simulink model "MultiEffectEvaporator_Forward"  (R2024a)
settings: Solver=VariableStepAuto  StartTime=0.0  StopTime=50  MaxStep=0.05  RelTol=1e-3
libraries: slpidlib x3
settings Model: Creator=tmlouw  LastModifiedBy=tmlouw

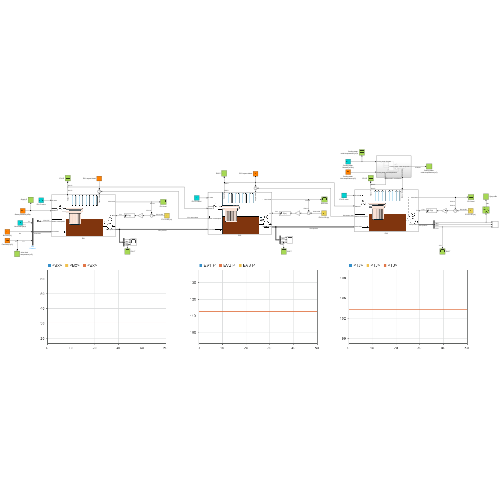
[thumbnail: Simulink's stored preview of the top-level diagram]
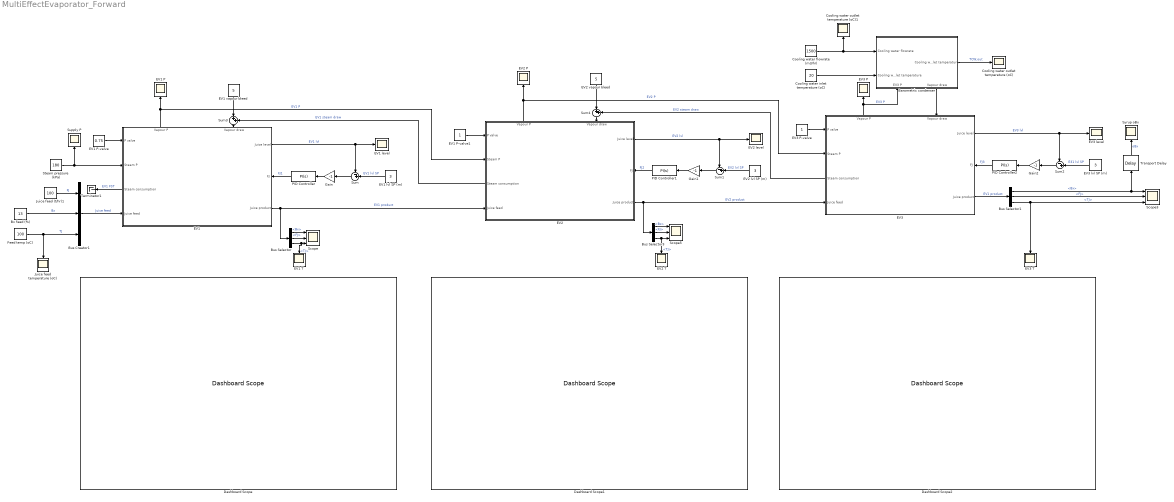
== system MultiEffectEvaporator_Forward ==
  Barometric condenser : Subsystem
      settings: PortSchema="{\"entries\":[{\"content\":{\"sides\":[{\"content\":{\"connectorIds\":[\"In1\",\"In2\"]},\"type\":\"ConnectorPlacement.EquallySpacedRectSide\",\"uuid\":\"e5056713-d8d2-44cb-a01c-60287b02fa20\"},{\"content\":{\"connectorIds\":[\"Out1\"],\"side\":\"RIGHT\"},\"type\":\"ConnectorPlacement.EquallySpacedRectSide\",\"uuid\":\"75a49828-ba17-4d10-97f5-6b462429e837\"},{\"content\":{\"side\":\"TOP\"},\"type\":\"ConnectorPlacement.EquallySpacedRectSide\",\"uuid\":\"088b5e1d-8405-4455-9e05-b28295e853da\"},{\"content\":{\"connectorIds\":[\"In3\",\"Out2\"],\"side\":\"BOTTOM\"},\"type\":\"ConnectorPlacement.EquallySpacedRectSide\",\"uuid\":\"29e66075-be5c-4fc5-8b50-76bd472c32b2\"}]},\"type\":\"ConnectorPlacement.EquallySpacedConnector\",\"uuid\":\"8d291cf1-31f4-4e5b-a130-7090ea448cc4\"}],\"packageUris\":[\"http://schema.mathworks.com/mf0/Connector/R2020b\"],\"version\":\"1.0\"}"
  Bus Creator1 : BusCreator  Inputs=3
  Bus Selector : BusSelector  OutputSignals=Bx,FJ,TJ
  Bus Selector1 : BusSelector  OutputSignals=Bx,FJ,TJ
  Bus Selector3 : BusSelector  OutputSignals=Bx,FJ,TJ
  Bx feed (%) : Constant  Value=13
  Cooling water flowrate (m3/hr) : Constant  Value=1500
  Cooling water inlet temperature (oC) : Constant  Value=20
  Cooling water outlet temperature (oC) : Scope
  Cooling water outlet temperature (oC)1 : Scope
  Dashboard Scope : DashboardScope
  Dashboard Scope1 : DashboardScope
  Dashboard Scope2 : DashboardScope
  EV1 : Subsystem
      settings: PortSchema="{\"entries\":[{\"content\":{\"sides\":[{\"content\":{\"connectorIds\":[\"In1\",\"In2\",\"Out4\",\"In3\"]},\"type\":\"ConnectorPlacement.EquallySpacedRectSide\",\"uuid\":\"23f23739-dcb1-4c27-bdfa-9a4fab3adfb4\"},{\"content\":{\"connectorIds\":[\"Out1\",\"In5\",\"Out2\"],\"side\":\"RIGHT\"},\"type\":\"ConnectorPlacement.EquallySpacedRectSide\",\"uuid\":\"36d72309-34f0-453c-bd76-e3ebc7b1c9b0\"},{\"content\":{\"connectorIds\":[\"Out3\",\"In4\"],\"side\":\"TOP\"},\"type\":\"ConnectorPlacement.EquallySpacedRectSide\",\"uuid\":\"a2c1fcb6-fda4-47d3-b526-f27431a4eb07\"},{\"content\":{\"side\":\"BOTTOM\"},\"type\":\"ConnectorPlacement.EquallySpacedRectSide\",\"uuid\":\"52c37164-7db0-4f32-b080-c60396f400a7\"}]},\"type\":\"ConnectorPlacement.EquallySpacedConnector\",\"uuid\":\"33257158-25c1-436c-a188-64f6424e9d36\"}],\"packageUris\":[\"http://schema.mathworks.com/mf0/Connector/R2020b\"],\"version\":\"1.0\"}"
      mask Display: image('MaskForward.png');
  EV1 P : Scope
  EV1 P-valve : Constant  Value=0.75
  EV1 P-valve1 : Constant
  EV1 T : Scope
  EV1 level : Scope
  EV1 lvl SP (m) : Constant  Value=3
  EV1 vapour bleed : Constant  Value=5
  EV2 : Subsystem
      settings: PortSchema="{\"entries\":[{\"content\":{\"sides\":[{\"content\":{\"connectorIds\":[\"In1\",\"In2\",\"Out4\",\"In3\"]},\"type\":\"ConnectorPlacement.EquallySpacedRectSide\",\"uuid\":\"23f23739-dcb1-4c27-bdfa-9a4fab3adfb4\"},{\"content\":{\"connectorIds\":[\"Out1\",\"In5\",\"Out2\"],\"side\":\"RIGHT\"},\"type\":\"ConnectorPlacement.EquallySpacedRectSide\",\"uuid\":\"36d72309-34f0-453c-bd76-e3ebc7b1c9b0\"},{\"content\":{\"connectorIds\":[\"Out3\",\"In4\"],\"side\":\"TOP\"},\"type\":\"ConnectorPlacement.EquallySpacedRectSide\",\"uuid\":\"a2c1fcb6-fda4-47d3-b526-f27431a4eb07\"},{\"content\":{\"side\":\"BOTTOM\"},\"type\":\"ConnectorPlacement.EquallySpacedRectSide\",\"uuid\":\"52c37164-7db0-4f32-b080-c60396f400a7\"}]},\"type\":\"ConnectorPlacement.EquallySpacedConnector\",\"uuid\":\"33257158-25c1-436c-a188-64f6424e9d36\"}],\"packageUris\":[\"http://schema.mathworks.com/mf0/Connector/R2020b\"],\"version\":\"1.0\"}"
      mask Display: image('MaskForward.png');
  EV2 P : Scope
  EV2 T : Scope
  EV2 level : Scope
  EV2 lvl SP (m) : Constant  Value=3
  EV2 vapour bleed : Constant  Value=5
  EV3 : Subsystem
      settings: PortSchema="{\"entries\":[{\"content\":{\"sides\":[{\"content\":{\"connectorIds\":[\"In1\",\"In2\",\"Out4\",\"In3\"]},\"type\":\"ConnectorPlacement.EquallySpacedRectSide\",\"uuid\":\"23f23739-dcb1-4c27-bdfa-9a4fab3adfb4\"},{\"content\":{\"connectorIds\":[\"Out1\",\"In5\",\"Out2\"],\"side\":\"RIGHT\"},\"type\":\"ConnectorPlacement.EquallySpacedRectSide\",\"uuid\":\"36d72309-34f0-453c-bd76-e3ebc7b1c9b0\"},{\"content\":{\"connectorIds\":[\"Out3\",\"In4\"],\"side\":\"TOP\"},\"type\":\"ConnectorPlacement.EquallySpacedRectSide\",\"uuid\":\"a2c1fcb6-fda4-47d3-b526-f27431a4eb07\"},{\"content\":{\"side\":\"BOTTOM\"},\"type\":\"ConnectorPlacement.EquallySpacedRectSide\",\"uuid\":\"52c37164-7db0-4f32-b080-c60396f400a7\"}]},\"type\":\"ConnectorPlacement.EquallySpacedConnector\",\"uuid\":\"33257158-25c1-436c-a188-64f6424e9d36\"}],\"packageUris\":[\"http://schema.mathworks.com/mf0/Connector/R2020b\"],\"version\":\"1.0\"}"
      mask Display: image('MaskForward.png');
  EV3 P : Scope
  EV3 P-valve : Constant
  EV3 T : Scope
  EV3 level : Scope
  EV3 lvl SP (m) : Constant  Value=3
  Feed temp (oC) : Constant  Value=100
  Gain : Gain  Gain=-1
  Gain1 : Gain  Gain=-1
  Gain2 : Gain  Gain=-1
  Juice feed temperature (oC) : Scope
  Juice feed (t/hr)1 : Constant  Value=100
  PID Controller : slpidlib/PID Controller  Controller=PI  Form=Parallel  TimeDomain=Continuous-time  UseExternalTs=off  SampleTime=-1  IntegratorMethod=Forward Euler  FilterMethod=Forward Euler  ControllerParametersSource=internal  P=1000  I=100  UseKiTs=off  D=0  UseExternalDerivativeSource=off  N=100  UseFilter=on  TunerSelectOption=Transfer Function Based (PID Tuner App)  InitialConditionSource=internal  InitialConditionForIntegrator=69.42  InitialConditionForFilter=0  DifferentiatorICPrevScaledInput=0  ExternalReset=none  TrackingMode=off  Kt=1  LimitOutput=on  SatLimitsSource=internal  UpperSaturationLimit=inf  LowerSaturationLimit=0  LinearizeAsGain=on  AntiWindupMode=none  Kb=1  LimitIntegrator=off  UpperIntegratorSaturationLimit=inf  LowerIntegratorSaturationLimit=-inf  POutMin=[]  POutMax=[]  IOutMin=[]  IOutMax=[]  DOutMin=[]  DOutMax=[]  NOutMin=[]  NOutMax=[]  SumOutMin=[]  SumOutMax=[]  SaturationOutMin=[]  SaturationOutMax=[]  PParamMin=[]  PParamMax=[]  IParamMin=[]  IParamMax=[]  DParamMin=[]  DParamMax=[]  NParamMin=[]  NParamMax=[]  KbParamMin=[]  KbParamMax=[]  KtParamMin=[]  KtParamMax=[]  KbOutMin=[]  KbOutMax=[]  KtOutMin=[]  KtOutMax=[]  IntegratorOutMin=[]  IntegratorOutMax=[]  FilterOutMin=[]  FilterOutMax=[]  SumI1OutMin=[]  SumI1OutMax=[]  SumI2OutMin=[]  SumI2OutMax=[]  SumI3OutMin=[]  SumI3OutMax=[]  SumI4OutMin=[]  SumI4OutMax=[]  SumDOutMin=[]  SumDOutMax=[]  DifferentiatorOutMin=[]  DifferentiatorOutMax=[]  FilterDiffOutCoefMin=[]  FilterDiffOutCoefMax=[]  ReciprocalOutMin=[]  ReciprocalOutMax=[]  SumDenOutMin=[]  SumDenOutMax=[]  SumNumOutMin=[]  SumNumOutMax=[]  DivideOutMin=[]  DivideOutMax=[]  UdiffTsProdOutMin=[]  UdiffTsProdOutMax=[]  NTsProdOutMin=[]  NTsProdOutMax=[]  UintegralTsProdOutMin=[]  UintegralTsProdOutMax=[]  UngainTsProdOutMin=[]  UngainTsProdOutMax=[]  ClampingZeroOutDataTypeStr=Inherit: Inherit via back propagation  ClampingZeroOutMin=[]  ClampingZeroOutMax=[]  FilterDenConstantOutDataTypeStr=Inherit: Inherit via back propagation  FilterDenConstantOutMin=[]  FilterDenConstantOutMax=[]  PCopyOutDataTypeStr=Inherit: Inherit via back propagation  PCopyOutMin=[]  PCopyOutMax=[]  NCopyOutDataTypeStr=Inherit: Inherit via back propagation  NCopyOutMin=[]  NCopyOutMax=[]  IntegratorContinuousStateAttributes=''  IntegratorStateMustResolveToSignalObject=off  IntegratorRTWStateStorageClass=Auto  FilterContinuousStateAttributes=''  FilterStateMustResolveToSignalObject=off  FilterRTWStateStorageClass=Auto  ParallelPVariant=InternalParameters  IdealPVariant=Disabled  IVariant=InternalParameters  DVariant=Disabled  IntegratorVariant=Continuous  SatVariant=Enabled  AWVariant=Passthrough  PCopyVariant=Disabled  TRVariant=Disabled  FdbkBlocksVariant=Forward  IdealPFdbkVariant=Disabled  SatFdbkVariant=Disabled  DerivativeFilterVariant=Disabled  NVariant=Disabled  NCopyVariant=Disabled_SignalSpec  FilterICVariant=Disabled  IntegratorICVariant=InternalICs  ExternalResetVariant=Disabled  TRSumVariant=Passthrough  SumFdbkVariant=Disabled  SumVariant=Sum_PI  TsampFilterVariant=InternalTs  TsampNgainVariant=Passthrough  TsampIntegralVariant=Disabled_SignalSpec  ExternalSaturationOutDataTypeStr=Inherit: Same as second input  DerivativeSourceVariant=Disabled
  PID Controller1 : slpidlib/PID Controller  Controller=PI  Form=Parallel  TimeDomain=Continuous-time  UseExternalTs=off  SampleTime=-1  IntegratorMethod=Forward Euler  FilterMethod=Forward Euler  ControllerParametersSource=internal  P=1000  I=100  UseKiTs=off  D=0  UseExternalDerivativeSource=off  N=100  UseFilter=on  TunerSelectOption=Transfer Function Based (PID Tuner App)  InitialConditionSource=internal  InitialConditionForIntegrator=43  InitialConditionForFilter=0  DifferentiatorICPrevScaledInput=0  ExternalReset=none  TrackingMode=off  Kt=1  LimitOutput=on  SatLimitsSource=internal  UpperSaturationLimit=inf  LowerSaturationLimit=0  LinearizeAsGain=on  AntiWindupMode=none  Kb=1  LimitIntegrator=off  UpperIntegratorSaturationLimit=inf  LowerIntegratorSaturationLimit=-inf  POutMin=[]  POutMax=[]  IOutMin=[]  IOutMax=[]  DOutMin=[]  DOutMax=[]  NOutMin=[]  NOutMax=[]  SumOutMin=[]  SumOutMax=[]  SaturationOutMin=[]  SaturationOutMax=[]  PParamMin=[]  PParamMax=[]  IParamMin=[]  IParamMax=[]  DParamMin=[]  DParamMax=[]  NParamMin=[]  NParamMax=[]  KbParamMin=[]  KbParamMax=[]  KtParamMin=[]  KtParamMax=[]  KbOutMin=[]  KbOutMax=[]  KtOutMin=[]  KtOutMax=[]  IntegratorOutMin=[]  IntegratorOutMax=[]  FilterOutMin=[]  FilterOutMax=[]  SumI1OutMin=[]  SumI1OutMax=[]  SumI2OutMin=[]  SumI2OutMax=[]  SumI3OutMin=[]  SumI3OutMax=[]  SumI4OutMin=[]  SumI4OutMax=[]  SumDOutMin=[]  SumDOutMax=[]  DifferentiatorOutMin=[]  DifferentiatorOutMax=[]  FilterDiffOutCoefMin=[]  FilterDiffOutCoefMax=[]  ReciprocalOutMin=[]  ReciprocalOutMax=[]  SumDenOutMin=[]  SumDenOutMax=[]  SumNumOutMin=[]  SumNumOutMax=[]  DivideOutMin=[]  DivideOutMax=[]  UdiffTsProdOutMin=[]  UdiffTsProdOutMax=[]  NTsProdOutMin=[]  NTsProdOutMax=[]  UintegralTsProdOutMin=[]  UintegralTsProdOutMax=[]  UngainTsProdOutMin=[]  UngainTsProdOutMax=[]  ClampingZeroOutDataTypeStr=Inherit: Inherit via back propagation  ClampingZeroOutMin=[]  ClampingZeroOutMax=[]  FilterDenConstantOutDataTypeStr=Inherit: Inherit via back propagation  FilterDenConstantOutMin=[]  FilterDenConstantOutMax=[]  PCopyOutDataTypeStr=Inherit: Inherit via back propagation  PCopyOutMin=[]  PCopyOutMax=[]  NCopyOutDataTypeStr=Inherit: Inherit via back propagation  NCopyOutMin=[]  NCopyOutMax=[]  IntegratorContinuousStateAttributes=''  IntegratorStateMustResolveToSignalObject=off  IntegratorRTWStateStorageClass=Auto  FilterContinuousStateAttributes=''  FilterStateMustResolveToSignalObject=off  FilterRTWStateStorageClass=Auto  ParallelPVariant=InternalParameters  IdealPVariant=Disabled  IVariant=InternalParameters  DVariant=Disabled  IntegratorVariant=Continuous  SatVariant=Enabled  AWVariant=Passthrough  PCopyVariant=Disabled  TRVariant=Disabled  FdbkBlocksVariant=Forward  IdealPFdbkVariant=Disabled  SatFdbkVariant=Disabled  DerivativeFilterVariant=Disabled  NVariant=Disabled  NCopyVariant=Disabled_SignalSpec  FilterICVariant=Disabled  IntegratorICVariant=InternalICs  ExternalResetVariant=Disabled  TRSumVariant=Passthrough  SumFdbkVariant=Disabled  SumVariant=Sum_PI  TsampFilterVariant=InternalTs  TsampNgainVariant=Passthrough  TsampIntegralVariant=Disabled_SignalSpec  ExternalSaturationOutDataTypeStr=Inherit: Same as second input  DerivativeSourceVariant=Disabled
  PID Controller2 : slpidlib/PID Controller  Controller=PI  Form=Parallel  TimeDomain=Continuous-time  UseExternalTs=off  SampleTime=-1  IntegratorMethod=Forward Euler  FilterMethod=Forward Euler  ControllerParametersSource=internal  P=1000  I=100  UseKiTs=off  D=0  UseExternalDerivativeSource=off  N=100  UseFilter=on  TunerSelectOption=Transfer Function Based (PID Tuner App)  InitialConditionSource=internal  InitialConditionForIntegrator=20.34  InitialConditionForFilter=0  DifferentiatorICPrevScaledInput=0  ExternalReset=none  TrackingMode=off  Kt=1  LimitOutput=on  SatLimitsSource=internal  UpperSaturationLimit=inf  LowerSaturationLimit=0  LinearizeAsGain=on  AntiWindupMode=none  Kb=1  LimitIntegrator=off  UpperIntegratorSaturationLimit=inf  LowerIntegratorSaturationLimit=-inf  POutMin=[]  POutMax=[]  IOutMin=[]  IOutMax=[]  DOutMin=[]  DOutMax=[]  NOutMin=[]  NOutMax=[]  SumOutMin=[]  SumOutMax=[]  SaturationOutMin=[]  SaturationOutMax=[]  PParamMin=[]  PParamMax=[]  IParamMin=[]  IParamMax=[]  DParamMin=[]  DParamMax=[]  NParamMin=[]  NParamMax=[]  KbParamMin=[]  KbParamMax=[]  KtParamMin=[]  KtParamMax=[]  KbOutMin=[]  KbOutMax=[]  KtOutMin=[]  KtOutMax=[]  IntegratorOutMin=[]  IntegratorOutMax=[]  FilterOutMin=[]  FilterOutMax=[]  SumI1OutMin=[]  SumI1OutMax=[]  SumI2OutMin=[]  SumI2OutMax=[]  SumI3OutMin=[]  SumI3OutMax=[]  SumI4OutMin=[]  SumI4OutMax=[]  SumDOutMin=[]  SumDOutMax=[]  DifferentiatorOutMin=[]  DifferentiatorOutMax=[]  FilterDiffOutCoefMin=[]  FilterDiffOutCoefMax=[]  ReciprocalOutMin=[]  ReciprocalOutMax=[]  SumDenOutMin=[]  SumDenOutMax=[]  SumNumOutMin=[]  SumNumOutMax=[]  DivideOutMin=[]  DivideOutMax=[]  UdiffTsProdOutMin=[]  UdiffTsProdOutMax=[]  NTsProdOutMin=[]  NTsProdOutMax=[]  UintegralTsProdOutMin=[]  UintegralTsProdOutMax=[]  UngainTsProdOutMin=[]  UngainTsProdOutMax=[]  ClampingZeroOutDataTypeStr=Inherit: Inherit via back propagation  ClampingZeroOutMin=[]  ClampingZeroOutMax=[]  FilterDenConstantOutDataTypeStr=Inherit: Inherit via back propagation  FilterDenConstantOutMin=[]  FilterDenConstantOutMax=[]  PCopyOutDataTypeStr=Inherit: Inherit via back propagation  PCopyOutMin=[]  PCopyOutMax=[]  NCopyOutDataTypeStr=Inherit: Inherit via back propagation  NCopyOutMin=[]  NCopyOutMax=[]  IntegratorContinuousStateAttributes=''  IntegratorStateMustResolveToSignalObject=off  IntegratorRTWStateStorageClass=Auto  FilterContinuousStateAttributes=''  FilterStateMustResolveToSignalObject=off  FilterRTWStateStorageClass=Auto  ParallelPVariant=InternalParameters  IdealPVariant=Disabled  IVariant=InternalParameters  DVariant=Disabled  IntegratorVariant=Continuous  SatVariant=Enabled  AWVariant=Passthrough  PCopyVariant=Disabled  TRVariant=Disabled  FdbkBlocksVariant=Forward  IdealPFdbkVariant=Disabled  SatFdbkVariant=Disabled  DerivativeFilterVariant=Disabled  NVariant=Disabled  NCopyVariant=Disabled_SignalSpec  FilterICVariant=Disabled  IntegratorICVariant=InternalICs  ExternalResetVariant=Disabled  TRSumVariant=Passthrough  SumFdbkVariant=Disabled  SumVariant=Sum_PI  TsampFilterVariant=InternalTs  TsampNgainVariant=Passthrough  TsampIntegralVariant=Disabled_SignalSpec  ExternalSaturationOutDataTypeStr=Inherit: Same as second input  DerivativeSourceVariant=Disabled
  Scope : Scope  NumInputPorts=3
  Scope3 : Scope  NumInputPorts=3
  Scope5 : Scope  NumInputPorts=3
  Steam pressure (kPa) : Constant  Value=180
  Sum : Sum  Inputs=-+|
  Sum1 : Sum  Inputs=-+|
  Sum2 : Sum  Inputs=-+|
  Sum3 : Sum  Inputs=|++
  Sum4 : Sum  Inputs=|++
  Supply P : Scope
  Syrup oBx : Scope
  Terminator1 : Terminator
  Transport Delay : TransportDelay  DelayTime=1/60
  wires:
  Gain/1 -> PID Controller/1
  PID Controller/1 -> EV1/5(FJ)  "FJ1"
  Sum/1 -> Gain/1
  EV1 lvl SP (m)/1 -> Sum/2  "EV1 lvl SP"
  EV1/4(Steam consumption) -> Terminator1/1  "EV1 FST"
  Bus Selector/2 -> Scope/2  "<FJ>"
  Bus Selector/1 -> Scope/1  "<Bx>"
  EV1 P-valve/1 -> EV1/1(P valve)
  EV1/2(Juice product) -> EV2/3(Juice feed), Bus Selector/1  "EV1 product"
  EV1 P-valve1/1 -> EV2/1(P valve)
  EV2/2(Juice product) -> EV3/3(Juice feed), Bus Selector3/1  "EV2 product"
  EV2/4(Steam consumption) -> Sum3/2  "EV1 steam draw"
  EV2 lvl SP (m)/1 -> Sum1/2  "EV2 lvl SP"
  Bus Selector3/1 -> Scope5/1  "<Bx>"
  Sum1/1 -> Gain1/1
  PID Controller1/1 -> EV2/5(FJ)  "FJ2"
  Gain1/1 -> PID Controller1/1
  Bus Selector3/2 -> Scope5/2  "<FJ>"
  Gain2/1 -> PID Controller2/1
  Bus Selector1/2 -> Scope3/2  "<FJ>"
  Bus Selector1/1 -> Scope3/1, Transport Delay/1  "<Bx>"
  EV3 lvl SP (m)/1 -> Sum2/2  "E31 lvl SP"
  PID Controller2/1 -> EV3/5(FJ)  "FJ3"
  EV3/2(Juice product) -> Bus Selector1/1  "EV1 product"
  Sum2/1 -> Gain2/1
  EV3/4(Steam consumption) -> Sum4/2  "EV2 steam draw"
  EV3 P-valve/1 -> EV3/1(P valve)
  EV1 vapour bleed/1 -> Sum3/1
  Sum3/1 -> EV1/4(Vapour draw)
  Sum4/1 -> EV2/4(Vapour draw)
  EV2 vapour bleed/1 -> Sum4/1
  Barometric condenser/2(Vapour draw) -> EV3/4(Vapour draw)
  Bx feed (%)/1 -> Bus Creator1/2  "Bx"
  Bus Creator1/1 -> EV1/3(Juice feed)  "Juice feed"
  Juice feed (t/hr)1/1 -> Bus Creator1/1  "FJ"
  Cooling water inlet temperature (oC)/1 -> Barometric condenser/2(Cooling water inlet temperature)
  Transport Delay/1 -> Syrup oBx/1  "oBx"
  Barometric condenser/1(Cooling water outlet temperature) -> Cooling water outlet temperature (oC)/1  "TCW,out"
  Cooling water flowrate (m3/hr)/1 -> Cooling water outlet temperature (oC)1/1, Barometric condenser/1(Cooling water flowrate)
  EV2/3(Vapour P) -> EV2 P/1, EV3/2(Steam P)  "EV2 P"
  EV1/3(Vapour P) -> EV1 P/1, EV2/2(Steam P)  "EV1 P"
  EV3/3(Vapour P) -> EV3 P/1, Barometric condenser/3(EV3 P)  "EV3 P"
  Steam pressure (kPa)/1 -> EV1/2(Steam P), Supply P/1
  Feed temp (oC)/1 -> Juice feed temperature (oC)/1, Bus Creator1/3  "TJ"
  EV2/1(Juice level) -> EV2 level/1, Sum1/1  "EV2 lvl"
  EV1/1(Juice level) -> EV1 level/1, Sum/1  "EV1 lvl"
  Bus Selector1/3 -> Scope3/3, EV3 T/1  "<TJ>"
  Bus Selector3/3 -> EV2 T/1, Scope5/3  "<TJ>"
  Bus Selector/3 -> EV1 T/1, Scope/3  "<TJ>"
  EV3/1(Juice level) -> Sum2/1, EV3 level/1  "EV3 lvl"

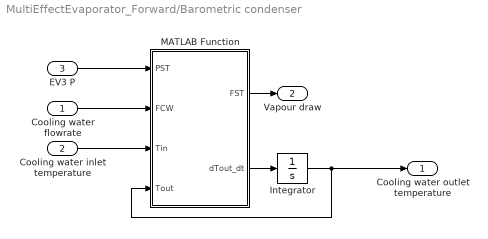
== system MultiEffectEvaporator_Forward/Barometric condenser ==
  Cooling water flowrate : Inport
  Cooling water inlet temperature : Inport  Port=2
  EV3 P : Inport  Port=3
  Integrator : Integrator  InitialCondition=27.85
  MATLAB Function : MATLAB Function  TreatAsAtomicUnit=on
  Cooling water outlet temperature : Outport
  Vapour draw : Outport  Port=2
  wires:
  MATLAB Function/2(dTout_dt) -> Integrator/1
  Cooling water flowrate/1 -> MATLAB Function/2(FCW)
  MATLAB Function/1(FST) -> Vapour draw/1
  Cooling water inlet temperature/1 -> MATLAB Function/3(Tin)
  Integrator/1 -> Cooling water outlet temperature/1, MATLAB Function/4(Tout)
  EV3 P/1 -> MATLAB Function/1(PST)

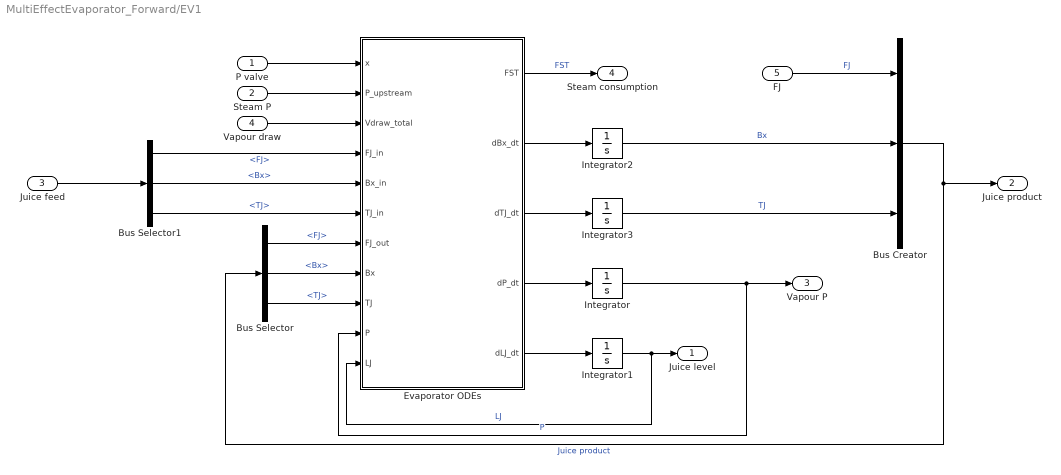
== system MultiEffectEvaporator_Forward/EV1 ==
  P valve : Inport
  Steam P : Inport  Port=2
  Juice feed : Inport  Port=3
  Vapour draw : Inport  Port=4
  FJ : Inport  Port=5
  Bus Creator : BusCreator  Inputs=3
  Bus Selector : BusSelector  OutputSignals=FJ,Bx,TJ
  Bus Selector1 : BusSelector  OutputSignals=FJ,Bx,TJ
  Evaporator ODEs : MATLAB Function  TreatAsAtomicUnit=on
  Integrator : Integrator  InitialCondition=135.79  LimitOutput=on  LowerSaturationLimit=0
  Integrator1 : Integrator  InitialCondition=3  LimitOutput=on  LowerSaturationLimit=0
  Integrator2 : Integrator  InitialCondition=18.73  UpperSaturationLimit=100  LowerSaturationLimit=0
  Integrator3 : Integrator  InitialCondition=108.72
  Juice level : Outport
  Juice product : Outport  Port=2
  Vapour P : Outport  Port=3
  Steam consumption : Outport  Port=4
  wires:
  Integrator2/1 -> Bus Creator/2  "Bx"
  Integrator/1 -> Evaporator ODEs/10(P), Vapour P/1  "P"
  Vapour draw/1 -> Evaporator ODEs/3(Vdraw_total)
  Bus Creator/1 -> Bus Selector/1, Juice product/1  "Juice product"
  Evaporator ODEs/4(dP_dt) -> Integrator/1
  Evaporator ODEs/1(FST) -> Steam consumption/1  "FST"
  Evaporator ODEs/3(dTJ_dt) -> Integrator3/1
  Bus Selector1/1 -> Evaporator ODEs/4(FJ_in)  "<FJ>"
  Integrator1/1 -> Juice level/1, Evaporator ODEs/11(LJ)  "LJ"
  P valve/1 -> Evaporator ODEs/1(x)
  Evaporator ODEs/5(dLJ_dt) -> Integrator1/1
  Evaporator ODEs/2(dBx_dt) -> Integrator2/1
  Bus Selector/2 -> Evaporator ODEs/8(Bx)  "<Bx>"
  Integrator3/1 -> Bus Creator/3  "TJ"
  Bus Selector/1 -> Evaporator ODEs/7(FJ_out)  "<FJ>"
  FJ/1 -> Bus Creator/1  "FJ"
  Bus Selector/3 -> Evaporator ODEs/9(TJ)  "<TJ>"
  Bus Selector1/3 -> Evaporator ODEs/6(TJ_in)  "<TJ>"
  Bus Selector1/2 -> Evaporator ODEs/5(Bx_in)  "<Bx>"
  Juice feed/1 -> Bus Selector1/1
  Steam P/1 -> Evaporator ODEs/2(P_upstream)

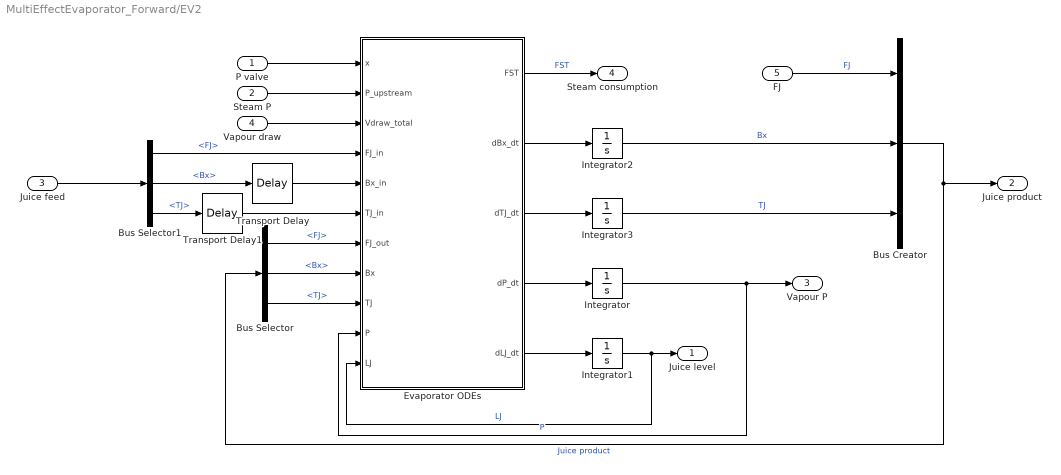
== system MultiEffectEvaporator_Forward/EV2 ==
  P valve : Inport
  Steam P : Inport  Port=2
  Juice feed : Inport  Port=3
  Vapour draw : Inport  Port=4
  FJ : Inport  Port=5
  Bus Creator : BusCreator  Inputs=3
  Bus Selector : BusSelector  OutputSignals=FJ,Bx,TJ
  Bus Selector1 : BusSelector  OutputSignals=FJ,Bx,TJ
  Evaporator ODEs : MATLAB Function  TreatAsAtomicUnit=on
  Integrator : Integrator  InitialCondition=112.38  LimitOutput=on  LowerSaturationLimit=0
  Integrator1 : Integrator  InitialCondition=3  LimitOutput=on  LowerSaturationLimit=0
  Integrator2 : Integrator  InitialCondition=30.23  UpperSaturationLimit=100  LowerSaturationLimit=0
  Integrator3 : Integrator  InitialCondition=103.3
  Transport Delay : TransportDelay  DelayTime=3/60  InitialOutput=18.73
  Transport Delay1 : TransportDelay  DelayTime=3/60  InitialOutput=108.72
  Juice level : Outport
  Juice product : Outport  Port=2
  Vapour P : Outport  Port=3
  Steam consumption : Outport  Port=4
  wires:
  Integrator2/1 -> Bus Creator/2  "Bx"
  Integrator/1 -> Evaporator ODEs/10(P), Vapour P/1  "P"
  Vapour draw/1 -> Evaporator ODEs/3(Vdraw_total)
  Bus Creator/1 -> Bus Selector/1, Juice product/1  "Juice product"
  Evaporator ODEs/4(dP_dt) -> Integrator/1
  Evaporator ODEs/1(FST) -> Steam consumption/1  "FST"
  Evaporator ODEs/3(dTJ_dt) -> Integrator3/1
  Bus Selector1/1 -> Evaporator ODEs/4(FJ_in)  "<FJ>"
  Integrator1/1 -> Juice level/1, Evaporator ODEs/11(LJ)  "LJ"
  P valve/1 -> Evaporator ODEs/1(x)
  Evaporator ODEs/5(dLJ_dt) -> Integrator1/1
  Evaporator ODEs/2(dBx_dt) -> Integrator2/1
  Bus Selector/2 -> Evaporator ODEs/8(Bx)  "<Bx>"
  Integrator3/1 -> Bus Creator/3  "TJ"
  Bus Selector/1 -> Evaporator ODEs/7(FJ_out)  "<FJ>"
  FJ/1 -> Bus Creator/1  "FJ"
  Bus Selector/3 -> Evaporator ODEs/9(TJ)  "<TJ>"
  Bus Selector1/3 -> Transport Delay1/1  "<TJ>"
  Bus Selector1/2 -> Transport Delay/1  "<Bx>"
  Juice feed/1 -> Bus Selector1/1
  Steam P/1 -> Evaporator ODEs/2(P_upstream)
  Transport Delay/1 -> Evaporator ODEs/5(Bx_in)
  Transport Delay1/1 -> Evaporator ODEs/6(TJ_in)

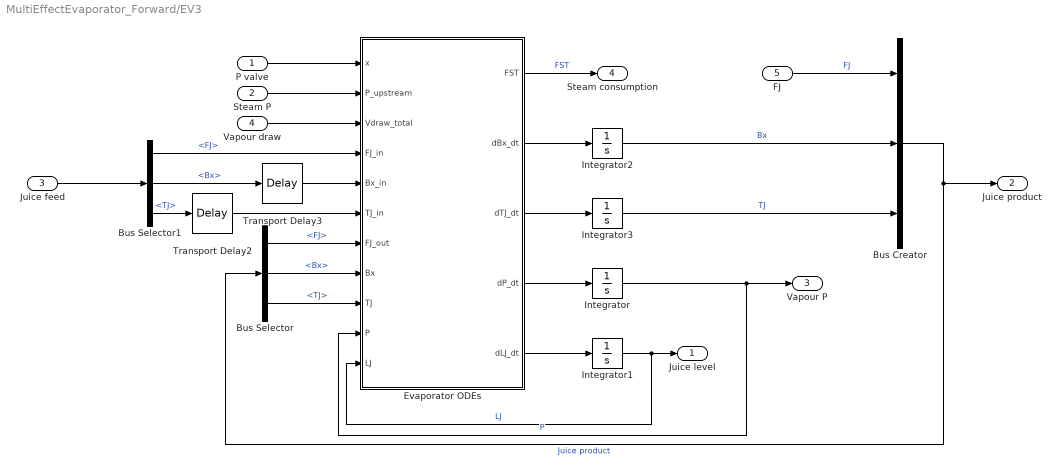
== system MultiEffectEvaporator_Forward/EV3 ==
  P valve : Inport
  Steam P : Inport  Port=2
  Juice feed : Inport  Port=3
  Vapour draw : Inport  Port=4
  FJ : Inport  Port=5
  Bus Creator : BusCreator  Inputs=3
  Bus Selector : BusSelector  OutputSignals=FJ,Bx,TJ
  Bus Selector1 : BusSelector  OutputSignals=FJ,Bx,TJ
  Evaporator ODEs : MATLAB Function  TreatAsAtomicUnit=on
  Integrator : Integrator  InitialCondition=95.4  LimitOutput=on  LowerSaturationLimit=0
  Integrator1 : Integrator  InitialCondition=3  LimitOutput=on  LowerSaturationLimit=0
  Integrator2 : Integrator  InitialCondition=63.9  UpperSaturationLimit=100  LowerSaturationLimit=0
  Integrator3 : Integrator  InitialCondition=98.77
  Transport Delay2 : TransportDelay  DelayTime=3/60  InitialOutput=103.3
  Transport Delay3 : TransportDelay  DelayTime=3/60  InitialOutput=30.23
  Juice level : Outport
  Juice product : Outport  Port=2
  Vapour P : Outport  Port=3
  Steam consumption : Outport  Port=4
  wires:
  Integrator2/1 -> Bus Creator/2  "Bx"
  Integrator/1 -> Evaporator ODEs/10(P), Vapour P/1  "P"
  Vapour draw/1 -> Evaporator ODEs/3(Vdraw_total)
  Bus Creator/1 -> Bus Selector/1, Juice product/1  "Juice product"
  Evaporator ODEs/4(dP_dt) -> Integrator/1
  Evaporator ODEs/1(FST) -> Steam consumption/1  "FST"
  Evaporator ODEs/3(dTJ_dt) -> Integrator3/1
  Bus Selector1/1 -> Evaporator ODEs/4(FJ_in)  "<FJ>"
  Integrator1/1 -> Juice level/1, Evaporator ODEs/11(LJ)  "LJ"
  P valve/1 -> Evaporator ODEs/1(x)
  Evaporator ODEs/5(dLJ_dt) -> Integrator1/1
  Evaporator ODEs/2(dBx_dt) -> Integrator2/1
  Bus Selector/2 -> Evaporator ODEs/8(Bx)  "<Bx>"
  Integrator3/1 -> Bus Creator/3  "TJ"
  Bus Selector/1 -> Evaporator ODEs/7(FJ_out)  "<FJ>"
  FJ/1 -> Bus Creator/1  "FJ"
  Bus Selector/3 -> Evaporator ODEs/9(TJ)  "<TJ>"
  Bus Selector1/3 -> Transport Delay2/1  "<TJ>"
  Bus Selector1/2 -> Transport Delay3/1  "<Bx>"
  Juice feed/1 -> Bus Selector1/1
  Steam P/1 -> Evaporator ODEs/2(P_upstream)
  Transport Delay3/1 -> Evaporator ODEs/5(Bx_in)
  Transport Delay2/1 -> Evaporator ODEs/6(TJ_in)

== matlab function MultiEffectEvaporator_Forward/EV2/Evaporator ODEs ==
  settings: updateMethod=CONTINUOUS  sampleTime=0.01
  data: x input; P_upstream input; Vdraw_total input; FST output; dBx_dt output; dTJ_dt output; dP_dt output; dLJ_dt output; FJ_in input; Bx_in input; TJ_in input; FJ_out input; Bx input; TJ input; P input; LJ input
function [FST, dBx_dt, dTJ_dt, dP_dt, dLJ_dt] = ODEs(x, P_upstream,Vdraw_total, FJ_in, Bx_in, TJ_in, FJ_out, Bx, TJ, P, LJ)
[FST, dBx_dt, dTJ_dt, dP_dt, dLJ_dt] = MultiEffectEvaporator_ODEs(x, P_upstream,Vdraw_total, FJ_in, Bx_in, TJ_in, FJ_out, Bx, TJ, P, LJ);

== matlab function MultiEffectEvaporator_Forward/EV3/Evaporator ODEs ==
  settings: updateMethod=CONTINUOUS  sampleTime=0.01
  data: x input; P_upstream input; Vdraw_total input; FST output; dBx_dt output; dTJ_dt output; dP_dt output; dLJ_dt output; FJ_in input; Bx_in input; TJ_in input; FJ_out input; Bx input; TJ input; P input; LJ input
function [FST, dBx_dt, dTJ_dt, dP_dt, dLJ_dt] = ODEs(x, P_upstream,Vdraw_total, FJ_in, Bx_in, TJ_in, FJ_out, Bx, TJ, P, LJ)
[FST, dBx_dt, dTJ_dt, dP_dt, dLJ_dt] = MultiEffectEvaporator_ODEs(x, P_upstream,Vdraw_total, FJ_in, Bx_in, TJ_in, FJ_out, Bx, TJ, P, LJ);

== matlab function MultiEffectEvaporator_Forward/Barometric condenser/MATLAB Function ==
  settings: updateMethod=CONTINUOUS
  data: PST input; FCW input; FST output; Tin input; Tout input; dTout_dt output
function [FST, dTout_dt] = Condenser(PST, FCW, Tin, Tout)
% Barometric condenser
% Inputs
%   PST (kPa):  pressure of steam entering the condenser
%   LCW (t/hr): cooling water flowrate
%   Tin (oC):   cooling water inlet temperature
%   Tout (oC):   cooling water outlet temperature

%% Parameters
U = 2500 *1e-6*3600; % (J/s.m2.oC) * (MJ/J) * (s/hr) = (MJ/hr.m2.oC): overall heat transfer coefficient
N = 400;             % (~): number of tubes
D = 25.4e-3;         % (m): tube diameter
L = 2.4;             % (m): tube length
A = N*pi*D*L;        % (m2): heat transfer area
V = N*pi*D^2/4*L;    % (m3): volume of cooling water in tubes
rho = 1;             % (t/m3): cooling water density
cp  = 4.187;         % (MJ/t.oC): cooling water heat capacity

%% Heat transfer 
% We assume heat transfer occurs between cooling water and condensed (saturated) water at PST
TST = fT_eq(PST);
LMTD = ( Tout - Tin) / log( (TST - Tin)/(TST - Tout) ); % (oC): log-mean temperature difference
Q = U*A*LMTD;                                     % (MJ/hr): heat transferred from steam

% Steam condensation rate
FST = Q/fdhvap(TST);

% Energy balance
dTout_dt = (FCW/V)*(Tin - Tout) + Q/(rho*V*cp);

end
%% Thermodynamics functions
% Saturation temperature (pure water)
function T_eq = fT_eq(P)
    T_eq =2188.8/(7.8656 - log10(P)) - 273.15;
end

% Heat of vaporisation (pure water)
function dhvap = fdhvap(T)
    Tr = (T + 273.15)/647.13;  % (~): reduced temperature of outgoing steam
    dhvap = 2889*(1-Tr)^(0.3199 - 0.212*Tr + 0.25795*Tr^2); % (MJ/t): heat of vapourisation
end

== matlab function MultiEffectEvaporator_Forward/EV1/Evaporator ODEs ==
  settings: updateMethod=CONTINUOUS  sampleTime=0.01
  data: x input; P_upstream input; Vdraw_total input; FST output; dBx_dt output; dTJ_dt output; dP_dt output; dLJ_dt output; FJ_in input; Bx_in input; TJ_in input; FJ_out input; Bx input; TJ input; P input; LJ input
function [FST, dBx_dt, dTJ_dt, dP_dt, dLJ_dt] = ODEs(x, P_upstream,Vdraw_total, FJ_in, Bx_in, TJ_in, FJ_out, Bx, TJ, P, LJ)
[FST, dBx_dt, dTJ_dt, dP_dt, dLJ_dt] = MultiEffectEvaporator_ODEs(x, P_upstream,Vdraw_total, FJ_in, Bx_in, TJ_in, FJ_out, Bx, TJ, P, LJ);
